simulink model "DTCIMD_30hp"  (R2014a)
settings: Solver=ode45  StartTime=0.0  StopTime=3.9  RelTol=1e-3
undefined symbols (not defined in the file): DiscIntNeverNeededParam, Lm, Lr, Ls1, Rs
libraries: powerlib x8, powerlib_meascontrol x6, simulink x1
settings Model: Creator=user  LastModifiedBy=Yugal
settings DataIOCC: SignalLoggingSaveFormat=ModelDataLogs
settings DebuggingCC: AlgebraicLoopMsg=none  UnderspecifiedInitializationDetection=Classic  MultiTaskDSMMsg=warning  MultiTaskCondExecSysMsg=none
settings RTWCC: IncludeERTFirstTime=on
settings SimscapeCC: EditingMode=Restricted

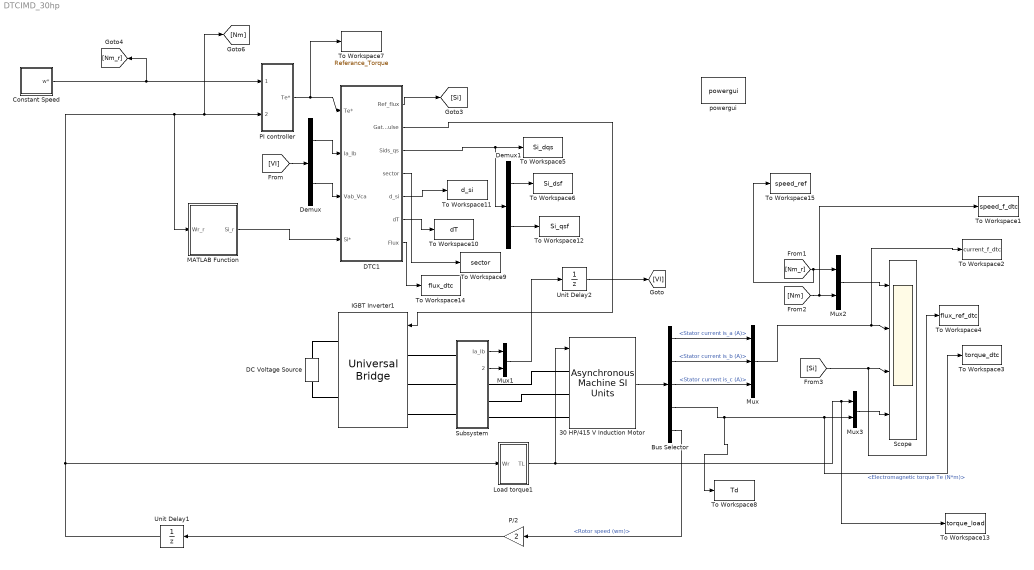
== system DTCIMD_30hp ==
  30 HP/415 V Induction Motor : powerlib/Machines/Asynchronous Machine SI Units  PresetModel=No  MechanicalLoad=Torque Tm  ShowDetailedParameters=on  RotorType=Squirrel-cage  ReferenceFrame=Stationary  Units=SI  MeasurementBus=off  NominalParameters=[30*746 415 50]  Stator=[Rs 0.001397]  Rotor=[0.249 0.001397]  Cage1=[ 0.022 0.226/377]  Cage2=[ 0.022 0.226/377]  Lm=0.0416  Mechanical=[0.305 0 2 ]  PolePairs=2  InitialConditions=[1 0 0 0 0 0 0 0]  SimulateSaturation=off  Saturation=[14.03593122, 27.81365428, 53.79336849, 72.68890987, 97.98006896, 148.6815601, 215.7428561, 302.9841135, 420.4778367 ; 230, 322, 414, 460, 506, 552, 598, 644, 690]  LoadFlowParameters=1492000  TsPowergui=0  TsBlock=-1  IterativeModel=Trapezoidal non iterative  Pmec=0
  Bus Selector : BusSelector  OutputSignals=Stator measurements.Stator current is_a (A),Stator measurements.Stator current is_b (A),Stator measurements.Stator current is_c (A),Mechanical.Electromagnetic torque Te (N*m),Mechanical.Rotor speed (wm)
  Constant Speed : Subsystem
  DC Voltage Source : powerlib/Electrical Sources/DC Voltage Source  Amplitude=560.44  Measurements=None
  DTC1 : Subsystem
  Demux : Demux  Outputs=2
  Demux1 : Demux  Outputs=2
  IGBT Inverter1 : powerlib/Power Electronics/Universal Bridge  Arms=3  SnubberResistance=1e5  SnubberCapacitance=inf  Device=MOSFET / Diodes  Ron=1e-3  Lon=0  ForwardVoltages="[  0  0  ]"  ForwardVoltage=0  GTOparameters=[ 10e-6 , 20e-6 ]  IGBTparameters=[ 1e-6 , 2e-6 ]  Measurements=None  Measurements_2=None  converterType=Rectifier
  Load torque1 : Subsystem
  MATLAB Function : MATLAB Function  TreatAsAtomicUnit=on
  Mux : Mux  Inputs=3
  Mux1 : Mux  Inputs=2
  Mux2 : Mux  Inputs=2
  Mux3 : Mux  Inputs=2
  P/2 : Gain  Gain=2
  PI controller : Subsystem  mask{Ki=1, Kp=90, Tlm=500, Ts=100e-6}
      mask prompts: Tlm "limit"; Ts "sampling time(sec)"
  Scope : Scope  NumInputPorts=4
      settings: TickLabels=on  TimeRange=3.4  YMin=70~-450~0.95~-900  YMax=260~450~1.05~400  MaxDataPoints=1000  Decimation=10
  Subsystem : Subsystem
  To Workspace1 : ToWorkspace  VariableName=speed_f_dtc  SaveFormat=Structure With Time  SampleTime=100e-6
  To Workspace10 : ToWorkspace  VariableName=dT  SaveFormat=Structure With Time  SampleTime=100e-6
  To Workspace11 : ToWorkspace  VariableName=d_si  SaveFormat=Structure With Time  SampleTime=100e-6
  To Workspace12 : ToWorkspace  VariableName=Si_qsf  SaveFormat=Structure With Time  SampleTime=100e-6
  To Workspace13 : ToWorkspace  VariableName=torque_load  SaveFormat=Structure With Time  SampleTime=100e-6
  To Workspace14 : ToWorkspace  VariableName=flux_dtc  SaveFormat=Structure With Time  SampleTime=100e-6
  To Workspace15 : ToWorkspace  VariableName=speed_ref  SaveFormat=Structure With Time  SampleTime=100e-6
  To Workspace2 : ToWorkspace  VariableName=current_f_dtc  SaveFormat=Structure With Time  SampleTime=100e-6
  To Workspace3 : ToWorkspace  VariableName=torque_dtc  SaveFormat=Structure With Time  SampleTime=100e-6
  To Workspace4 : ToWorkspace  VariableName=flux_ref_dtc  SaveFormat=Structure With Time  SampleTime=100e-6
  To Workspace5 : ToWorkspace  VariableName=Si_dqs  SaveFormat=Structure With Time  SampleTime=100e-6
  To Workspace6 : ToWorkspace  VariableName=Si_dsf  SaveFormat=Structure With Time  SampleTime=100e-6
  To Workspace7 : ToWorkspace  VariableName=Referance_Torque  SaveFormat=Structure With Time  SampleTime=100e-6
  To Workspace8 : ToWorkspace  VariableName=Td  SaveFormat=Structure With Time  SampleTime=100e-6
  To Workspace9 : ToWorkspace  VariableName=sector  SaveFormat=Structure With Time  SampleTime=100e-6
  Unit Delay1 : UnitDelay  SampleTime=100e-6
  Unit Delay2 : UnitDelay  SampleTime=10e-6
  powergui : powerlib/powergui  Priority=1  SimulationMode=Discrete  SolverType=Backward Euler  SampleTime=10e-6  frequency=60  SPID=off  DisableSnubberDevices=off  DisableRonSwitches=off  DisableVfSwitches=off  SwTol=0  Interpol=off  DisplayEquations=off  Ts=0  methode=off  frequencyindice=50  Pbase=100e6  ErrMax=1e-4  Iterations=50  UnitsV=kV  UnitsW=MW  FunctionMessages=off  echomessages=off  HookPort=off  EnableUseOfTLC=off  x0status=blocks  RestoreLinks=warning  ResistiveCurrentMeasurement=off  Frange=[0:2:500]  Ylog=off  Xlog=on  ShowGrid=off  save=off  variable=ZData  structure=torque_dtc  ZoomFFT=off  StartTime=2  cycles=1  DisplayStyle=1  fundamental=50  FreqAxis=off  MaxFrequency=10000  frequencyindicesteady=1  RmsSteady=1  display=off
  wires:
  30 HP/415 V Induction Motor/1 -> Bus Selector/1
  [Nm_r] -> To Workspace15/1, Mux2/1
  [Nm] -> To Workspace1/1, Mux2/2
  Bus Selector/3 -> Mux/3  "<Stator current is_c (A)>"
  Bus Selector/2 -> Mux/2  "<Stator current is_b (A)>"
  Bus Selector/1 -> Mux/1  "<Stator current is_a (A)>"
  DTC1/1(Ref_flux) -> [Si]
  [Si] -> To Workspace4/1, Scope/3
  Load torque1/1(TL) -> 30 HP/415 V Induction Motor/1, To Workspace13/1, Mux3/1
  Bus Selector/4 -> To Workspace8/1, To Workspace3/1, Mux3/2  "<Electromagnetic torque Te (N*m)>"
  PI controller/1(Te*) -> To Workspace7/1, DTC1/1(Te*)
  Subsystem/1(Ia_Ib) -> Mux1/1
  Subsystem/2(Vba_Vac) -> Mux1/2
  [VI] -> Demux/1
  Demux/2 -> DTC1/3(Vab_Vca)
  Demux/1 -> DTC1/2(Ia_Ib)
  Unit Delay1/1 -> Load torque1/1(Wr), MATLAB Function/1(Wr_r), PI controller/2(Wm), [Nm]
  Constant Speed/1(w*) -> PI controller/1(Wm*), [Nm_r]
  DTC1/2(Gate Pulse) -> IGBT Inverter1/1
  Mux2/1 -> Scope/1
  Mux3/1 -> Scope/4
  Mux/1 -> To Workspace2/1, Scope/2
  P/2/1 -> Unit Delay1/1
  Bus Selector/5 -> P/2/1  "<Rotor speed (wm)>"
  Unit Delay2/1 -> [VI]
  Mux1/1 -> Unit Delay2/1
  DTC1/5(d_si) -> To Workspace11/1
  DTC1/6(dT) -> To Workspace10/1
  DTC1/3(Sids_qs) -> Demux1/1, To Workspace5/1
  DTC1/4(sector) -> To Workspace9/1
  Demux1/1 -> To Workspace6/1
  Demux1/2 -> To Workspace12/1
  DTC1/7(Flux) -> To Workspace14/1
  MATLAB Function/1(Si_r) -> DTC1/4(Si*)
  connections:
  30 HP/415 V Induction Motor/LConn1 -- Subsystem/RConn1
  30 HP/415 V Induction Motor/LConn3 -- Subsystem/RConn3
  30 HP/415 V Induction Motor/LConn2 -- Subsystem/RConn2
  IGBT Inverter1/LConn3 -- Subsystem/LConn3
  IGBT Inverter1/LConn2 -- Subsystem/LConn2
  IGBT Inverter1/LConn1 -- Subsystem/LConn1
  DC Voltage Source/RConn1 -- IGBT Inverter1/RConn1
  DC Voltage Source/LConn1 -- IGBT Inverter1/RConn2

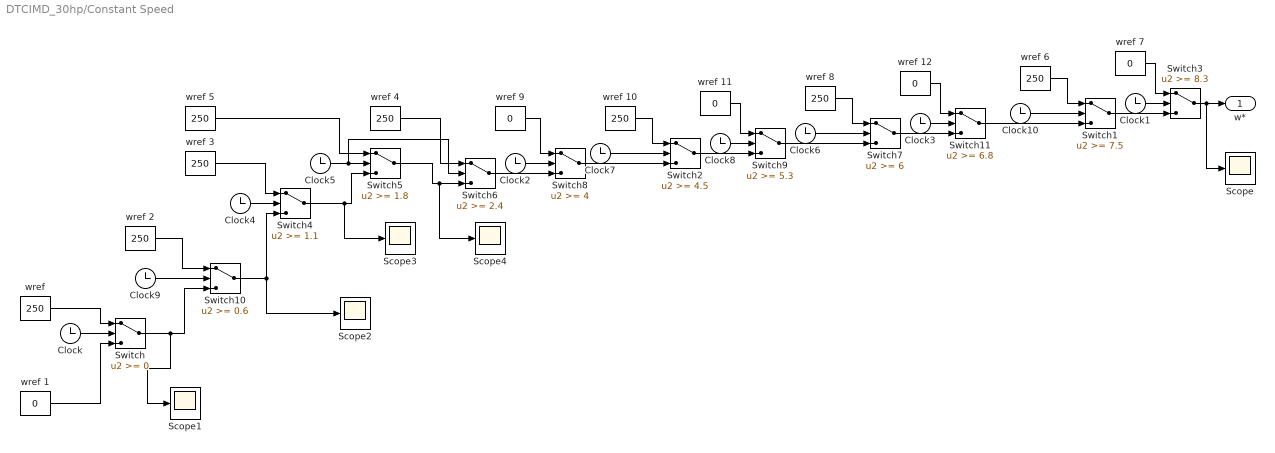
== system DTCIMD_30hp/Constant Speed ==
  Clock{,1..10} (11 alike) : Clock
      settings: Decimation=2
  Scope{,1..4} (5 alike) : Scope
      Scope1 settings: SaveName=ScopeData2
      Scope2 settings: YMin=-300  YMax=300  SaveName=ScopeData3
      Scope3 settings: SaveName=ScopeData4
      Scope4 settings: SaveName=ScopeData5
  Switch : Switch  SaturateOnIntegerOverflow=on  InputSameDT=on
  Switch1 : Switch  Threshold=7.5  SaturateOnIntegerOverflow=on  InputSameDT=on
  Switch10 : Switch  Threshold=0.6  SaturateOnIntegerOverflow=on  InputSameDT=on
  Switch11 : Switch  Threshold=6.8  SaturateOnIntegerOverflow=on  InputSameDT=on
  Switch2 : Switch  Threshold=4.5  SaturateOnIntegerOverflow=on  InputSameDT=on
  Switch3 : Switch  Threshold=8.3  SaturateOnIntegerOverflow=on  InputSameDT=on
  Switch4 : Switch  Threshold=1.1  SaturateOnIntegerOverflow=on  InputSameDT=on
  Switch5 : Switch  Threshold=1.8  SaturateOnIntegerOverflow=on  InputSameDT=on
  Switch6 : Switch  Threshold=2.4  SaturateOnIntegerOverflow=on  InputSameDT=on
  Switch7 : Switch  Threshold=6  SaturateOnIntegerOverflow=on  InputSameDT=on
  Switch8 : Switch  Threshold=4  SaturateOnIntegerOverflow=on  InputSameDT=on
  Switch9 : Switch  Threshold=5.3  SaturateOnIntegerOverflow=on  InputSameDT=on
  wref {,2..6,8,10} (8 alike) : Constant  Value=250
  wref {1,7,9,11..12} (5 alike) : Constant  Value=0
  w* : Outport
  wires:
  wref 1/1 -> Switch/3
  Clock/1 -> Switch/2
  "wref "/1 -> Switch/1
  Clock4/1 -> Switch4/2
  wref 3/1 -> Switch4/1
  Switch4/1 -> Scope3/1, Switch5/3
  Switch5/1 -> Scope4/1, Switch6/3
  Clock5/1 -> Switch6/2, Switch5/2
  wref 4/1 -> Switch6/1
  wref 5/1 -> Switch5/1
  Switch10/1 -> Switch4/3, Scope2/1
  Switch6/1 -> Switch8/3
  wref 9/1 -> Switch8/1
  Clock2/1 -> Switch8/2
  Switch8/1 -> Switch2/3
  Clock7/1 -> Switch2/2
  wref 10/1 -> Switch2/1
  Switch2/1 -> Switch9/3
  Clock8/1 -> Switch9/2
  wref 11/1 -> Switch9/1
  Switch/1 -> Scope1/1, Switch10/3
  Clock9/1 -> Switch10/2
  wref 2/1 -> Switch10/1
  Switch11/1 -> Switch1/3
  Clock10/1 -> Switch1/2
  wref 6/1 -> Switch1/1
  Switch1/1 -> Switch3/3
  Clock1/1 -> Switch3/2
  wref 7/1 -> Switch3/1
  Clock6/1 -> Switch7/2
  wref 8/1 -> Switch7/1
  Switch7/1 -> Switch11/3
  Clock3/1 -> Switch11/2
  wref 12/1 -> Switch11/1
  Switch9/1 -> Switch7/3
  Switch3/1 -> Scope/1, w*/1

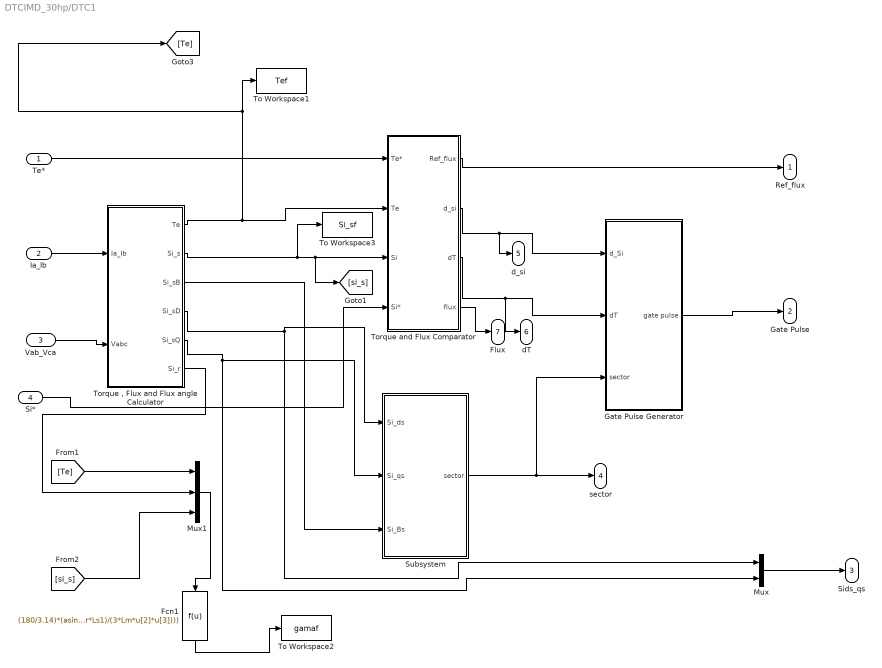
== system DTCIMD_30hp/DTC1 ==
  Te* : Inport
  Ia_Ib : Inport  Port=2
  Vab_Vca : Inport  Port=3
  Si* : Inport  Port=4
  Fcn1 : Fcn  Expr=(180/3.14)*(asin((u[1]*Lr*Ls1)/(3*Lm*u[2]*u[3])))
  Gate Pulse Generator : Subsystem
  Mux : Mux  Inputs=2
  Mux1 : Mux  Inputs=3
  Subsystem : Subsystem
  To Workspace1 : ToWorkspace  VariableName=Tef  SaveFormat=Structure With Time  SampleTime=100e-6
  To Workspace2 : ToWorkspace  VariableName=gamaf  SaveFormat=Structure With Time  SampleTime=100e-6
  To Workspace3 : ToWorkspace  VariableName=Si_sf  SaveFormat=Structure With Time  SampleTime=100e-6
  "Torque , Flux and Flux angle Calculator" : Subsystem
  Torque and Flux Comparator : Subsystem
  Ref_flux : Outport
  Gate Pulse : Outport  Port=2
  Sids_qs : Outport  Port=3
  sector : Outport  Port=4
  d_si : Outport  Port=5
  dT : Outport  Port=6
  Flux : Outport  Port=7
  wires:
  Si*/1 -> Torque and Flux Comparator/4(Si*)
  Te*/1 -> Torque and Flux Comparator/1(Te*)
  "Torque , Flux and Flux angle Calculator"/1(Te) -> To Workspace1/1, [Te], Torque and Flux Comparator/2(Te)
  Gate Pulse Generator/1(gate pulse) -> Gate Pulse/1
  Torque and Flux Comparator/3(dT) -> dT/1, Gate Pulse Generator/2(dT)
  Torque and Flux Comparator/2(d_si) -> d_si/1, Gate Pulse Generator/1(d_Si)
  Ia_Ib/1 -> "Torque , Flux and Flux angle Calculator"/1(Ia_Ib)
  Torque and Flux Comparator/1(Ref_flux) -> Ref_flux/1
  Vab_Vca/1 -> "Torque , Flux and Flux angle Calculator"/2(Vabc)
  "Torque , Flux and Flux angle Calculator"/4(Si_sD) -> Subsystem/1(Si_ds), Mux/1
  "Torque , Flux and Flux angle Calculator"/5(Si_sQ) -> Mux/2, Subsystem/2(Si_qs)
  "Torque , Flux and Flux angle Calculator"/3(Si_sB) -> Subsystem/3(Si_Bs)
  Subsystem/1(sector) -> sector/1, Gate Pulse Generator/3(sector)
  "Torque , Flux and Flux angle Calculator"/2(Si_s) -> To Workspace3/1, [si_s], Torque and Flux Comparator/3(Si)
  Mux/1 -> Sids_qs/1
  [Te] -> Mux1/1
  "Torque , Flux and Flux angle Calculator"/6("Si_r ") -> Mux1/2
  [si_s] -> Mux1/3
  Mux1/1 -> Fcn1/1
  Fcn1/1 -> To Workspace2/1
  Torque and Flux Comparator/4(flux) -> Flux/1

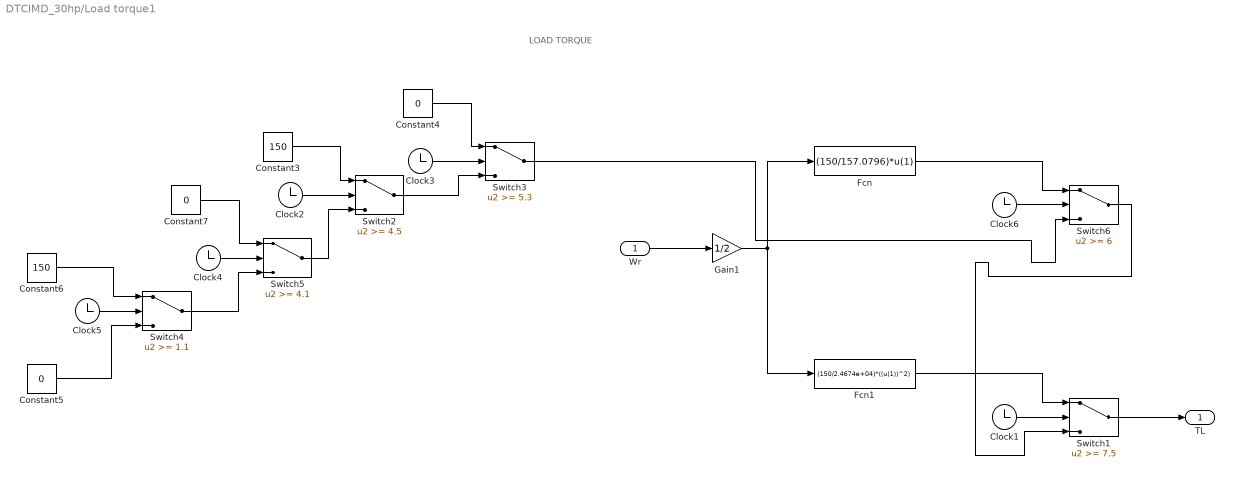
== system DTCIMD_30hp/Load torque1 ==
  note: LOAD TORQUE
  Wr : Inport
  Clock{1..6} (6 alike) : Clock
  Constant3 : Constant  Value=150
  Constant4 : Constant  Value=0
  Constant5 : Constant  Value=0
  Constant6 : Constant  Value=150
  Constant7 : Constant  Value=0
  Fcn : Fcn  Expr=(150/157.0796)*u(1)
  Fcn1 : Fcn  Expr=(150/2.4674e+04)*((u(1))^2)
  Gain1 : Gain  Gain=1/2
  Switch1 : Switch  Threshold=7.5
  Switch2 : Switch  Threshold=4.5
  Switch3 : Switch  Threshold=5.3
  Switch4 : Switch  Threshold=1.1
  Switch5 : Switch  Threshold=4.1
  Switch6 : Switch  Threshold=6
  TL : Outport
  wires:
  Switch5/1 -> Switch2/3
  Clock2/1 -> Switch2/2
  Switch2/1 -> Switch3/3
  Clock3/1 -> Switch3/2
  Constant3/1 -> Switch2/1
  Constant4/1 -> Switch3/1
  Wr/1 -> Gain1/1
  Gain1/1 -> Fcn/1, Fcn1/1
  Constant5/1 -> Switch4/3
  Constant6/1 -> Switch4/1
  Switch4/1 -> Switch5/3
  Clock4/1 -> Switch5/2
  Constant7/1 -> Switch5/1
  Clock5/1 -> Switch4/2
  Clock6/1 -> Switch6/2
  Fcn/1 -> Switch6/1
  Switch3/1 -> Switch6/3
  Clock1/1 -> Switch1/2
  Fcn1/1 -> Switch1/1
  Switch6/1 -> Switch1/3
  Switch1/1 -> TL/1

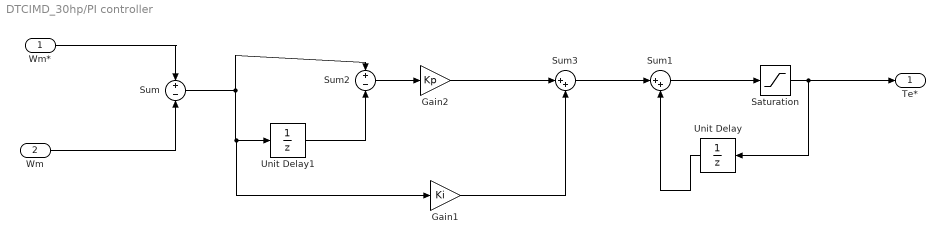
== system DTCIMD_30hp/PI controller ==
  Wm* : Inport
  Wm : Inport  Port=2
  Gain1 : Gain  Gain=Ki
  Gain2 : Gain  Gain=Kp
  Saturation : Saturate  UpperLimit=Tlm  LowerLimit=-Tlm
  Sum : Sum  Inputs=+-
  Sum1 : Sum  Inputs=|++
  Sum2 : Sum  Inputs=+-
  Sum3 : Sum  Inputs=|++
  Unit Delay : UnitDelay  SampleTime=Ts
  Unit Delay1 : UnitDelay  SampleTime=Ts
  Te* : Outport
  wires:
  Sum2/1 -> Gain2/1
  Gain2/1 -> Sum3/1
  Gain1/1 -> Sum3/2
  Sum1/1 -> Saturation/1
  Unit Delay/1 -> Sum1/2
  Saturation/1 -> Te*/1, Unit Delay/1
  Wm*/1 -> Sum/1
  Sum/1 -> Gain1/1, Unit Delay1/1, Sum2/1
  Unit Delay1/1 -> Sum2/2
  Sum3/1 -> Sum1/1
  Wm/1 -> Sum/2

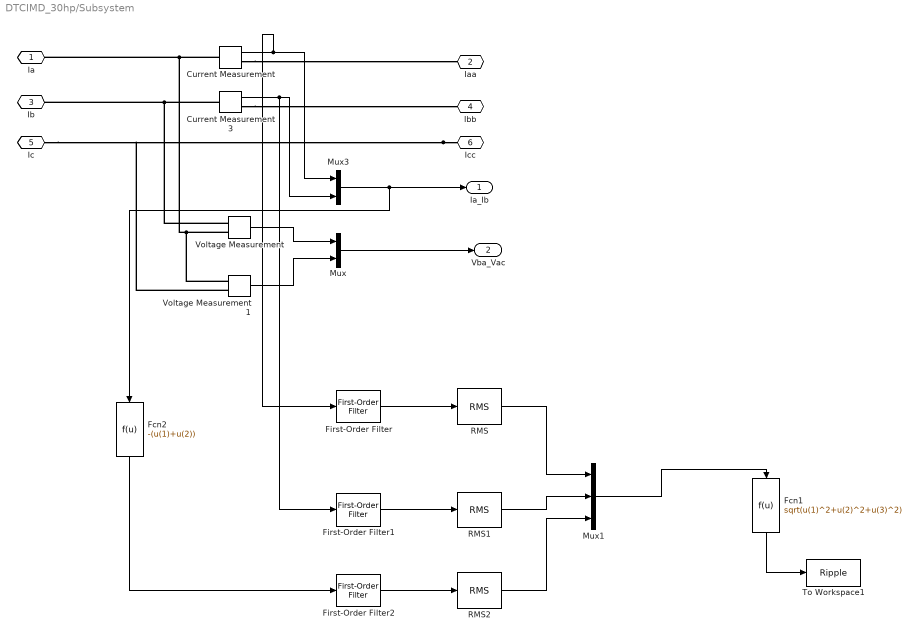
== system DTCIMD_30hp/Subsystem ==
  Current Measurement : powerlib/Measurements/Current Measurement  PhasorSimulation=off  OutputType=Complex  PSBequivalent=0
  Current Measurement3 : powerlib/Measurements/Current Measurement  PhasorSimulation=off  OutputType=Complex  PSBequivalent=0
  Fcn1 : Fcn  Expr=sqrt(u(1)^2+u(2)^2+u(3)^2)
  Fcn2 : Fcn  Expr=-(u(1)+u(2))
  First-Order Filter : powerlib_meascontrol/Filters/First-Order Filter  FilterType=Highpass  Tc=2e-3  Ts=0  Initialize=on  Vac_Init=[0, 0, 50]  Vdc_Init=0  PlotResponse=off  FreqRange="[0,  200,  1]"
  First-Order Filter1 : powerlib_meascontrol/Filters/First-Order Filter  FilterType=Highpass  Tc=2e-3  Ts=0  Initialize=on  Vac_Init=[0, 0, 50]  Vdc_Init=0  PlotResponse=off  FreqRange="[0,  200,  1]"
  First-Order Filter2 : powerlib_meascontrol/Filters/First-Order Filter  FilterType=Highpass  Tc=2e-3  Ts=0  Initialize=on  Vac_Init=[0, 0, 50]  Vdc_Init=0  PlotResponse=off  FreqRange="[0,  200,  1]"
  Mux : Mux  Inputs=2
  Mux1 : Mux  Inputs=3
  Mux3 : Mux  Inputs=2
  RMS : powerlib_meascontrol/Measurements/RMS  TrueRMS=on  Freq=60  RMSInit=120  Ts=0
  RMS1 : powerlib_meascontrol/Measurements/RMS  TrueRMS=on  Freq=60  RMSInit=120  Ts=0
  RMS2 : powerlib_meascontrol/Measurements/RMS  TrueRMS=on  Freq=60  RMSInit=120  Ts=0
  To Workspace1 : ToWorkspace  VariableName=Ripple  SaveFormat=Structure With Time  SampleTime=100e-6
  Voltage Measurement : powerlib/Measurements/Voltage Measurement  PhasorSimulation=off  OutputType=Complex  PSBequivalent=0
  Voltage Measurement1 : powerlib/Measurements/Voltage Measurement  PhasorSimulation=off  OutputType=Complex  PSBequivalent=0
  Ia : PMIOPort  Port=1  Side=Left
  Iaa : PMIOPort  Port=2  Side=Right
  Ib : PMIOPort  Port=3  Side=Left
  Ibb : PMIOPort  Port=4  Side=Right
  Ic : PMIOPort  Port=5  Side=Right
  Icc : PMIOPort  Port=6  Side=Left
  Ia_Ib : Outport
  Vba_Vac : Outport  Port=2
  wires:
  Mux/1 -> Vba_Vac/1
  Current Measurement3/1 -> Mux3/2, First-Order Filter1/1
  Current Measurement/1 -> First-Order Filter/1, Mux3/1
  Voltage Measurement1/1 -> Mux/2
  Voltage Measurement/1 -> Mux/1
  First-Order Filter/1 -> RMS/1
  Fcn2/1 -> First-Order Filter2/1
  First-Order Filter1/1 -> RMS1/1
  First-Order Filter2/1 -> RMS2/1
  RMS/1 -> Mux1/1
  RMS1/1 -> Mux1/2
  RMS2/1 -> Mux1/3
  Mux1/1 -> Fcn1/1
  Fcn1/1 -> To Workspace1/1
  Mux3/1 -> Fcn2/1, Ia_Ib/1
  connections:
  Current Measurement/RConn1 -- Iaa/RConn1
  Voltage Measurement/LConn1 -- Current Measurement3/LConn1 -- Ib/RConn1
  Current Measurement3/RConn1 -- Ibb/RConn1
  Voltage Measurement/LConn2 -- Voltage Measurement1/LConn1 -- Current Measurement/LConn1 -- Ia/RConn1
  Icc/RConn1 -- Ic/RConn1 -- Voltage Measurement1/LConn2

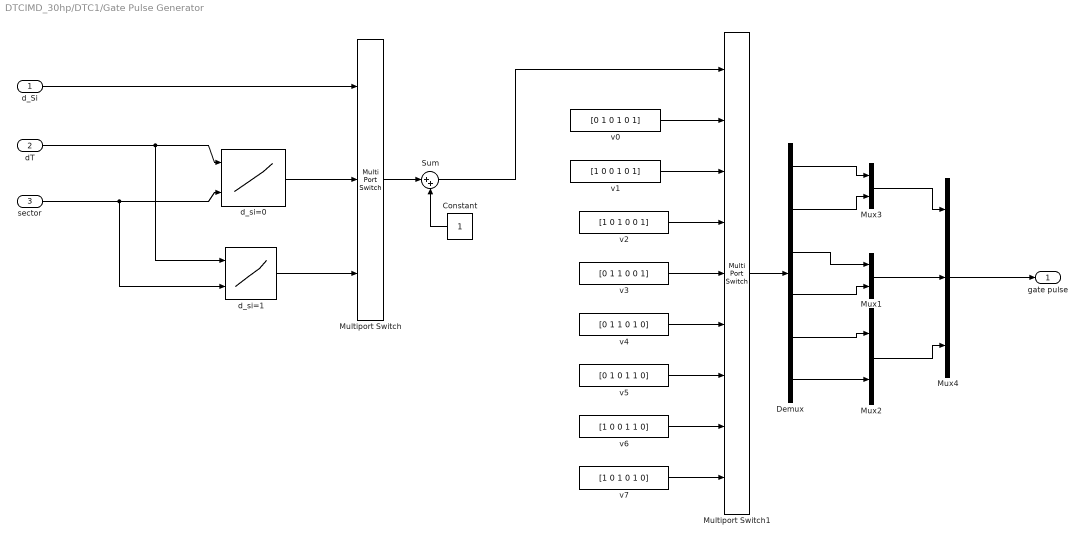
== system DTCIMD_30hp/DTC1/Gate Pulse Generator ==
  d_Si : Inport
  dT : Inport  Port=2
  sector : Inport  Port=3
  Constant : Constant
  Demux : Demux  Outputs=6
  Multiport Switch : MultiPortSwitch  DataPortOrder=Zero-based contiguous  Inputs=2  DiagnosticForDefault=None
  Multiport Switch1 : MultiPortSwitch  Inputs=8  DiagnosticForDefault=None
  Mux1 : Mux  Inputs=2
  Mux2 : Mux  Inputs=2
  Mux3 : Mux  Inputs=2
  Mux4 : Mux  Inputs=3
  Sum : Sum  Inputs=|++
  d_si=0 : Lookup_n-D  BreakpointsForDimension1=[-1;0;1]  BreakpointsForDimension2=[1;2;3;4;5;6]  BreakpointsForDimension3=[5, 7]  Table=[5 6 1 2 3 4;7 0 7 0 7 0;3 4 5 6 1 2]  RndMeth=Simplest  InputSameDT=on
  d_si=1 : Lookup_n-D  BreakpointsForDimension1=[-1;0;1]  BreakpointsForDimension2=[1;2;3;4;5;6]  BreakpointsForDimension3=[5, 7]  Table=[6 1 2 3 4 5;0 7 0 7 0 7;2 3 4 5 6 1;]  OutDataTypeStr=Inherit: Inherit from 'Table data'  RndMeth=Simplest  InputSameDT=on
  v0 : Constant  Value=[0 1 0 1 0 1]
  v1 : Constant  Value=[1 0 0 1 0 1]
  v2 : Constant  Value=[1 0 1 0 0 1]
  v3 : Constant  Value=[0 1 1 0 0 1]
  v4 : Constant  Value=[0 1 1 0 1 0]
  v5 : Constant  Value=[0 1 0 1 1 0]
  v6 : Constant  Value=[1 0 0 1 1 0]
  v7 : Constant  Value=[1 0 1 0 1 0]
  gate pulse : Outport
  wires:
  v0/1 -> Multiport Switch1/2
  d_Si/1 -> Multiport Switch/1
  dT/1 -> d_si=1/1, d_si=0/1
  sector/1 -> d_si=1/2, d_si=0/2
  v7/1 -> Multiport Switch1/9
  v3/1 -> Multiport Switch1/5
  v6/1 -> Multiport Switch1/8
  v4/1 -> Multiport Switch1/6
  v5/1 -> Multiport Switch1/7
  v2/1 -> Multiport Switch1/4
  Sum/1 -> Multiport Switch1/1
  Multiport Switch/1 -> Sum/1
  Constant/1 -> Sum/2
  v1/1 -> Multiport Switch1/3
  Multiport Switch1/1 -> Demux/1
  Demux/3 -> Mux1/1
  Demux/4 -> Mux1/2
  Demux/1 -> Mux3/1
  Demux/2 -> Mux3/2
  Demux/6 -> Mux2/2
  Demux/5 -> Mux2/1
  Mux3/1 -> Mux4/1
  Mux1/1 -> Mux4/2
  Mux2/1 -> Mux4/3
  Mux4/1 -> gate pulse/1
  d_si=1/1 -> Multiport Switch/3
  d_si=0/1 -> Multiport Switch/2

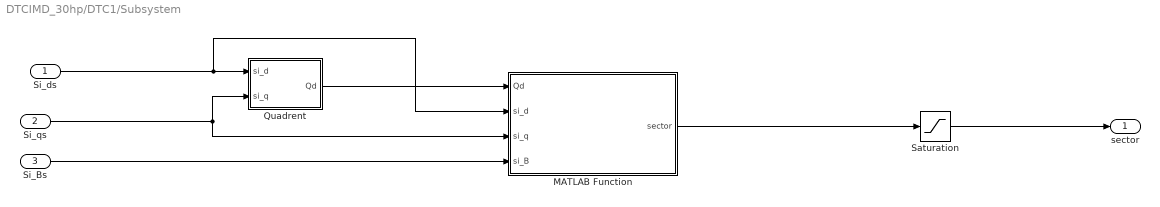
== system DTCIMD_30hp/DTC1/Subsystem ==
  Si_ds : Inport
  Si_qs : Inport  Port=2
  Si_Bs : Inport  Port=3
  MATLAB Function : MATLAB Function  TreatAsAtomicUnit=on
  Quadrent : MATLAB Function  TreatAsAtomicUnit=on
  Saturation : Saturate  UpperLimit=6  LowerLimit=1
  sector : Outport
  wires:
  MATLAB Function/1(sector) -> Saturation/1
  Saturation/1 -> sector/1
  Si_Bs/1 -> MATLAB Function/4(si_B)
  Si_ds/1 -> MATLAB Function/2(si_d), Quadrent/1(si_d)
  Quadrent/1(Qd) -> MATLAB Function/1(Qd)
  Si_qs/1 -> Quadrent/2(si_q), MATLAB Function/3(si_q)

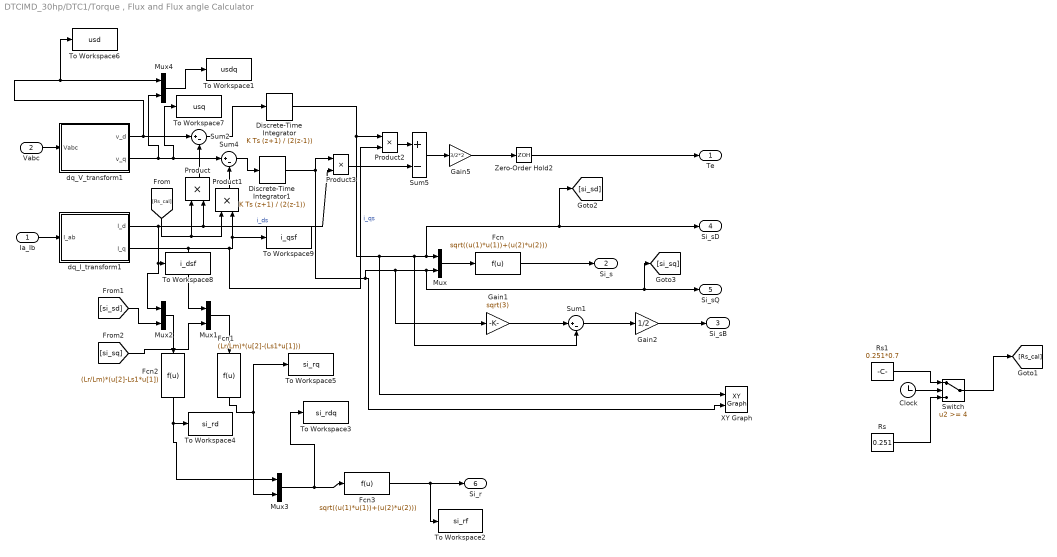
== system DTCIMD_30hp/DTC1/Torque , Flux and Flux angle Calculator ==
  Ia_Ib : Inport
  Vabc : Inport  Port=2
  Clock : Clock
      settings: Decimation=2
  Discrete-Time Integrator : DiscreteIntegrator  IntegratorMethod=Integration: Trapezoidal  SampleTime=100e-6  ICPrevOutput=DiscIntNeverNeededParam  ICPrevScaledInput=DiscIntNeverNeededParam
  Discrete-Time Integrator1 : DiscreteIntegrator  IntegratorMethod=Integration: Trapezoidal  SampleTime=100e-6  ICPrevOutput=DiscIntNeverNeededParam  ICPrevScaledInput=DiscIntNeverNeededParam
  Fcn : Fcn  Expr=sqrt((u(1)*u(1))+(u(2)*u(2)))
  Fcn1 : Fcn  Expr=(Lr/Lm)*(u[2]-(Ls1*u[1]))
  Fcn2 : Fcn  Expr=(Lr/Lm)*(u[2]-Ls1*u[1])
  Fcn3 : Fcn  Expr=sqrt((u(1)*u(1))+(u(2)*u(2)))
  Gain1 : Gain  Gain=sqrt(3)  SaturateOnIntegerOverflow=on  OutDataTypeStr=Inherit: Same as input  ParamDataTypeStr=Inherit: Same as input
  Gain2 : Gain  Gain=1/2  SaturateOnIntegerOverflow=on  OutDataTypeStr=Inherit: Same as input  ParamDataTypeStr=Inherit: Same as input
  Gain5 : Gain  Gain=3/2*2  SaturateOnIntegerOverflow=on  OutDataTypeStr=Inherit: Same as input  ParamDataTypeStr=Inherit: Same as input
  Mux{,1..4} (5 alike) : Mux  Inputs=2
  Product : Product
  Product1 : Product
  Product2 : Product  SaturateOnIntegerOverflow=on  OutDataTypeStr=Inherit: Same as first input
  Product3 : Product  SaturateOnIntegerOverflow=on  OutDataTypeStr=Inherit: Same as first input
  Rs : Constant  Value=0.251
  Rs1 : Constant  Value=0.251*0.7
  Sum1 : Sum  Inputs=|+-  SaturateOnIntegerOverflow=on
  Sum2 : Sum  Inputs=|+-  SaturateOnIntegerOverflow=on
  Sum4 : Sum  Inputs=|+-  SaturateOnIntegerOverflow=on
  Sum5 : Sum  Inputs=+-  SaturateOnIntegerOverflow=on
  Switch : Switch  Threshold=4  SaturateOnIntegerOverflow=on  InputSameDT=on
  To Workspace1 : ToWorkspace  VariableName=usdq  SaveFormat=Structure With Time  SampleTime=100e-6
  To Workspace2 : ToWorkspace  VariableName=si_rf  SaveFormat=Structure With Time  SampleTime=100e-6
  To Workspace3 : ToWorkspace  VariableName=si_rdq  SaveFormat=Structure With Time  SampleTime=100e-6
  To Workspace4 : ToWorkspace  VariableName=si_rd  SaveFormat=Structure With Time  SampleTime=100e-6
  To Workspace5 : ToWorkspace  VariableName=si_rq  SaveFormat=Structure With Time  SampleTime=100e-6
  To Workspace6 : ToWorkspace  VariableName=usd  SaveFormat=Structure With Time  SampleTime=100e-6
  To Workspace7 : ToWorkspace  VariableName=usq  SaveFormat=Structure With Time  SampleTime=100e-6
  To Workspace8 : ToWorkspace  VariableName=i_dsf  SaveFormat=Structure With Time  SampleTime=100e-6
  To Workspace9 : ToWorkspace  VariableName=i_qsf  SaveFormat=Structure With Time  SampleTime=100e-6
  XY Graph : simulink/Sinks/XY Graph  xmin=-1.5  xmax=1.5  ymin=-1.5  ymax=1.5  st=-1
  Zero-Order Hold2 : ZeroOrderHold  SampleTime=100e-6
  dq_I_transform1 : Subsystem
  dq_V_transform1 : Subsystem
  Te : Outport
  Si_s : Outport  Port=2
  Si_sB : Outport  Port=3
  Si_sD : Outport  Port=4
  Si_sQ : Outport  Port=5
  "Si_r " : Outport  Port=6
  wires:
  Product/1 -> Sum2/2
  Ia_Ib/1 -> dq_I_transform1/1(I_ab)
  Sum2/1 -> Discrete-Time Integrator/1
  Product1/1 -> Sum4/2
  Sum4/1 -> Discrete-Time Integrator1/1
  Product2/1 -> Sum5/1
  Product3/1 -> Sum5/2
  Sum5/1 -> Gain5/1
  Gain5/1 -> Zero-Order Hold2/1
  Zero-Order Hold2/1 -> Te/1
  Mux/1 -> Fcn/1
  Fcn/1 -> Si_s/1
  Gain1/1 -> Sum1/1
  Sum1/1 -> Gain2/1
  Gain2/1 -> Si_sB/1
  Vabc/1 -> dq_V_transform1/1(Vabc)
  Discrete-Time Integrator1/1 -> Product3/1, Gain1/1, [si_sq], Si_sQ/1, Mux/2, XY Graph/2
  Discrete-Time Integrator/1 -> Sum1/2, [si_sd], Si_sD/1, Mux/1, XY Graph/1, Product2/1
  dq_V_transform1/1(v_d) -> Mux4/1, To Workspace6/1, Sum2/1
  dq_V_transform1/2(v_q) -> Mux4/2, To Workspace7/1, Sum4/1
  dq_I_transform1/1(I_d) -> To Workspace8/1, Mux2/1, Product/2, Product3/2  "i_ds"
  dq_I_transform1/2(I_q) -> Mux1/1, To Workspace9/1, Product1/2, Product2/2  "i_qs"
  Fcn2/1 -> To Workspace4/1, Mux3/1
  Fcn1/1 -> Mux3/2, To Workspace5/1
  [si_sd] -> Mux2/2
  Mux2/1 -> Fcn2/1
  [si_sq] -> Mux1/2
  Mux1/1 -> Fcn1/1
  Mux3/1 -> To Workspace3/1, Fcn3/1
  Fcn3/1 -> To Workspace2/1, "Si_r "/1
  Mux4/1 -> To Workspace1/1
  Rs/1 -> Switch/3
  Clock/1 -> Switch/2
  Rs1/1 -> Switch/1
  Switch/1 -> [Rs_cal]
  [Rs_cal] -> Product1/1, Product/1

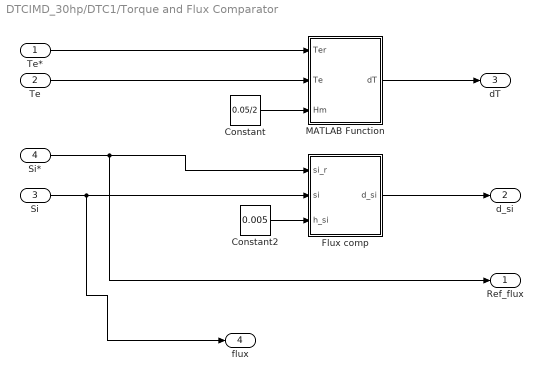
== system DTCIMD_30hp/DTC1/Torque and Flux Comparator ==
  Te* : Inport
  Te : Inport  Port=2
  Si : Inport  Port=3
  Si* : Inport  Port=4
  Constant : Constant  Value=0.05/2
  Constant2 : Constant  Value=0.005
  Flux comp : MATLAB Function  TreatAsAtomicUnit=on
  MATLAB Function : MATLAB Function  TreatAsAtomicUnit=on
  Ref_flux : Outport
  d_si : Outport  Port=2
  dT : Outport  Port=3
  flux : Outport  Port=4
  wires:
  Si*/1 -> Ref_flux/1, Flux comp/1(si_r)
  Flux comp/1(d_si) -> d_si/1
  Te/1 -> MATLAB Function/2(Te)
  Si/1 -> flux/1, Flux comp/2(si)
  Constant/1 -> MATLAB Function/3(Hm)
  Te*/1 -> MATLAB Function/1(Ter)
  MATLAB Function/1(dT) -> dT/1
  Constant2/1 -> Flux comp/3(h_si)

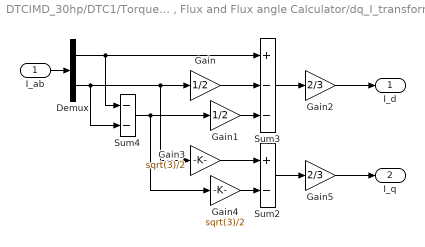
== system DTCIMD_30hp/DTC1/Torque , Flux and Flux angle Calculator/dq_I_transform1 ==
  I_ab : Inport
  Demux : Demux  Outputs=2
  Gain : Gain  Gain=1/2  SaturateOnIntegerOverflow=on  OutDataTypeStr=Inherit: Same as input  ParamDataTypeStr=Inherit: Same as input
  Gain1 : Gain  Gain=1/2  SaturateOnIntegerOverflow=on  OutDataTypeStr=Inherit: Same as input  ParamDataTypeStr=Inherit: Same as input
  Gain2 : Gain  Gain=2/3  SaturateOnIntegerOverflow=on  OutDataTypeStr=Inherit: Same as input  ParamDataTypeStr=Inherit: Same as input
  Gain3 : Gain  Gain=sqrt(3)/2  SaturateOnIntegerOverflow=on  OutDataTypeStr=Inherit: Same as input  ParamDataTypeStr=Inherit: Same as input
  Gain4 : Gain  Gain=sqrt(3)/2  SaturateOnIntegerOverflow=on  OutDataTypeStr=Inherit: Same as input  ParamDataTypeStr=Inherit: Same as input
  Gain5 : Gain  Gain=2/3  SaturateOnIntegerOverflow=on  OutDataTypeStr=Inherit: Same as input  ParamDataTypeStr=Inherit: Same as input
  Sum2 : Sum  Inputs=+-  SaturateOnIntegerOverflow=on  InputSameDT=on  OutDataTypeStr=Inherit: Same as first input
  Sum3 : Sum  Inputs=+--  SaturateOnIntegerOverflow=on  InputSameDT=on  OutDataTypeStr=Inherit: Same as first input
  Sum4 : Sum  Inputs=--  SaturateOnIntegerOverflow=on  InputSameDT=on  OutDataTypeStr=Inherit: Same as first input
  I_d : Outport
  I_q : Outport  Port=2
  wires:
  Sum2/1 -> Gain5/1
  Gain4/1 -> Sum2/2
  Gain3/1 -> Sum2/1
  Sum3/1 -> Gain2/1
  Sum4/1 -> Gain4/1, Gain1/1
  Gain/1 -> Sum3/2
  Gain1/1 -> Sum3/3
  Demux/2 -> Sum4/2, Gain/1, Gain3/1
  Demux/1 -> Sum4/1, Sum3/1
  I_ab/1 -> Demux/1
  Gain5/1 -> I_q/1
  Gain2/1 -> I_d/1

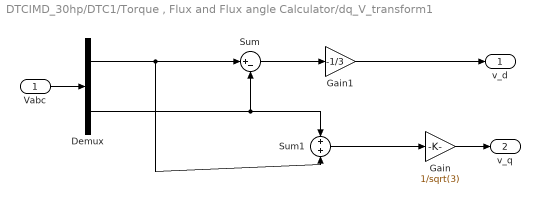
== system DTCIMD_30hp/DTC1/Torque , Flux and Flux angle Calculator/dq_V_transform1 ==
  Vabc : Inport
  Demux : Demux  Outputs=2
  Gain : Gain  Gain=1/sqrt(3)
  Gain1 : Gain  Gain=-1/3
  Sum : Sum  Inputs=|+-
  Sum1 : Sum
  v_d : Outport
  v_q : Outport  Port=2
  wires:
  Vabc/1 -> Demux/1
  Demux/1 -> Sum/1, Sum1/2
  Sum/1 -> Gain1/1
  Gain1/1 -> v_d/1
  Gain/1 -> v_q/1
  Demux/2 -> Sum/2, Sum1/1
  Sum1/1 -> Gain/1

== matlab function DTCIMD_30hp/DTC1/Torque and Flux Comparator/Flux comp ==
  data: si_r input; d_si output; si input; h_si input
function d_si = fcn(si_r,si,h_si)
d_si=1;
if (si_r-si)>h_si
    d_si=1;
elseif (( (si_r-si)>-h_si) && ((si_r-si)<h_si) && d_si==1)
    d_si=1;
elseif  ((si_r-si)<-h_si)
    d_si=0;
elseif ( ((si_r-si)>-h_si) && ((si_r-si)<h_si) && d_si==0)
    d_si=0;
end

== matlab function DTCIMD_30hp/MATLAB Function ==
  data: Si_r output; Wr_r input
function Si_r = fcn(Wr_r)
if Wr_r<2*pi*50
    Si_r=1;
else
   
    Si_r=2*pi*50/Wr_r;
    
end
end

== matlab function DTCIMD_30hp/DTC1/Subsystem/MATLAB Function ==
  data: Qd input; sector output; si_d input; si_q input; si_B input
function sector = fcn(Qd,si_d,si_q,si_B)
sector = 1;
if Qd == 1 && si_d>0 && si_B<=0
    sector = 1;
elseif Qd == 1 && si_d>=0 && si_B>0
    sector = 2;
elseif Qd == 2 && (abs(si_q/si_d)>=0.5774) && si_d<0 && si_B>0
    sector = 3; 
elseif Qd == 2 && (abs(si_q/si_d)<0.5774) && si_d<0 && si_B>0
    sector = 4;
elseif Qd == 3 && si_d<0 && si_B>=0
    sector = 4; 
elseif Qd == 3 && si_d<=0 && si_B<0
    sector = 5;
elseif Qd == 4 && (abs(si_q/si_d)>=0.5774) && si_d>0 && si_B<0
    sector = 6;    
elseif Qd == 4 && (abs(si_q/si_d)<0.5774) && si_d>0 && si_B<0
    sector = 1; 
end

== matlab function DTCIMD_30hp/DTC1/Torque and Flux Comparator/MATLAB Function ==
  data: Ter input; dT output; Te input; Hm input
function dT = fcn( Ter,Te,Hm )
dT=0;
if ((Ter-Te)> Hm)
    dT=1;
elseif ((Ter-Te)>0 && (Ter-Te)<Hm && dT==1)
    dT=1;
elseif ((Ter-Te)<-Hm)
    dT=-1;
elseif ((Ter-Te)>-Hm && (Ter-Te)<0 && dT==-1)
    dT=-1;
elseif ((Ter-Te)>0 && (Ter-Te)<Hm && dT==-1)
    dT=0;
elseif ((Ter-Te)>-Hm && (Ter-Te)<0 && dT==1)
    dT=0;
end

end

== matlab function DTCIMD_30hp/DTC1/Subsystem/Quadrent ==
  data: si_d input; Qd output; si_q input
function Qd = fcn(si_d,si_q)
Qd=1;
if si_d>=0 && si_q>=0
    Qd=1;
elseif si_d<0 && si_q>0
    Qd=2;
elseif si_d<0 && si_q<0
    Qd=3;
elseif si_d>0 && si_q<0
    Qd=4;
end

end
